simulink model "Hardware"  (R2020b)
settings: Solver=VariableStepAuto  StartTime=0.0  StopTime=10.0  RelTol=1e-3
libraries: arduinolib x4
settings Model: Creator=99003186  LastModifiedBy=99003178

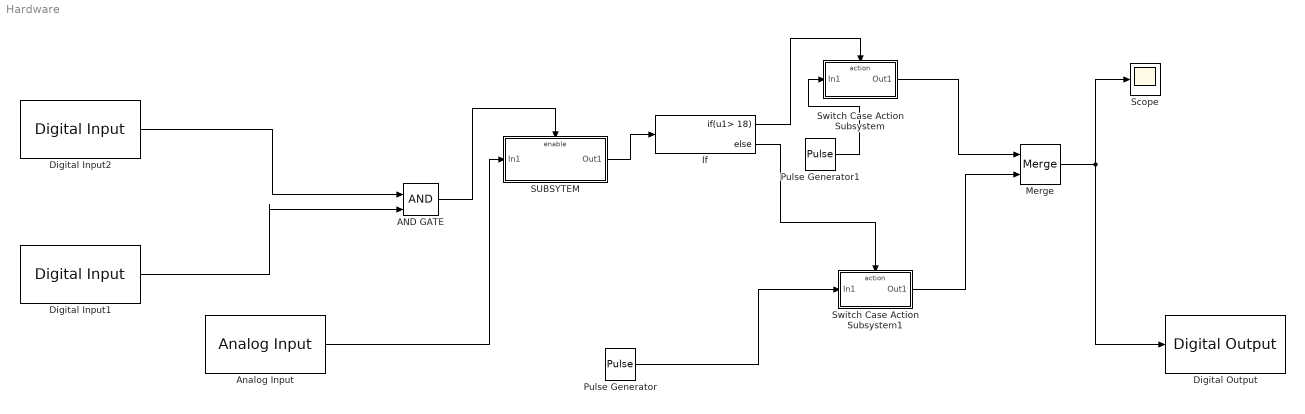
== system Hardware ==
  AND GATE : Logic  IconShape=distinctive  AllPortsSameDT=off  OutDataTypeStr=boolean
  Analog Input : arduinolib/Analog Input  pinNumber=4  ReadResultsOnly=off  ConversionTriggerSource=Software  ExternalTriggerType=uint32( 0 )  OutputDataType=uint16  EnableConversionCompleteNotify=off  EnableOuputStatus=off  SampleTime=-1  blockPlatform=arduino
  Digital Input1 : arduinolib/Digital Input  pinNumber=12  mode=Default  Direction=input  SampleTime=0.1  blockPlatform=arduino
  Digital Input2 : arduinolib/Digital Input  pinNumber=8  mode=Default  Direction=input  SampleTime=0.1  blockPlatform=arduino
  Digital Output : arduinolib/Digital Output  pinNumber=9  Direction=output  blockPlatform=arduino
  If : If  IfExpression=u1> 18
  Merge : Merge
  Pulse Generator : DiscretePulseGenerator  PulseType=Time based  Period=10  PulseWidth=5
  Pulse Generator1 : DiscretePulseGenerator  PulseType=Time based  Period=10  PulseWidth=5
  SUBSYTEM : Subsystem
  Scope : Scope
  Switch Case Action Subsystem : Subsystem  TreatAsAtomicUnit=on
  Switch Case Action Subsystem1 : Subsystem  TreatAsAtomicUnit=on
  wires:
  Switch Case Action Subsystem1/1(Out1) -> Merge/2
  If/2 -> Switch Case Action Subsystem1/Action
  AND GATE/1 -> SUBSYTEM/Enable
  Pulse Generator/1 -> Switch Case Action Subsystem1/1(In1)
  If/1 -> Switch Case Action Subsystem/Action
  Switch Case Action Subsystem/1(Out1) -> Merge/1
  Digital Input2/1 -> AND GATE/1
  Pulse Generator1/1 -> Switch Case Action Subsystem/1(In1)
  SUBSYTEM/1(Out1) -> If/1
  Analog Input/1 -> SUBSYTEM/1(In1)
  Digital Input1/1 -> AND GATE/2
  Merge/1 -> Scope/1, Digital Output/1

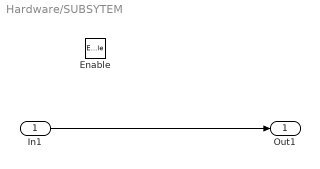
== system Hardware/SUBSYTEM ==
  In1 : Inport
  Enable : EnablePort
  Out1 : Outport
  wires:
  In1/1 -> Out1/1

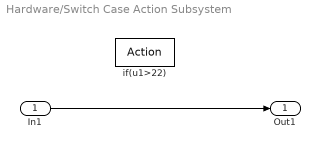
== system Hardware/Switch Case Action Subsystem ==
  In1 : Inport
  if(u1>22) : ActionPort  ActionPortLabel=if(u1> 18)
  Out1 : Outport
  wires:
  In1/1 -> Out1/1

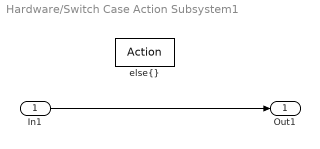
== system Hardware/Switch Case Action Subsystem1 ==
  In1 : Inport
  "else{}" : ActionPort  ActionPortLabel=else
  Out1 : Outport
  wires:
  In1/1 -> Out1/1
